simulink model "ULMPC_ES_multi_sine"  (R2020a)
settings: Solver=ode1  StartTime=0.0  StopTime=1900  FixedStep=1/600  RelTol=1e-3
values from neighbouring files (symbols this model uses):
  alpha_IC = [60000;10000]    [initial_run.m]
  amp = 0.03*[60000;10000]    [initial_run.m]
  freq = [(2*pi)/(5*Tr); (2*pi)/(4*Tr)]    [initial_run.m]
  gain_es = -[0.01;0.007]*30000    [initial_run.m]
  i_max = 0.85    [initial_run.m]
  Q = 16    [initial_run.m]
  R_weight = 10    [initial_run.m]
  Tr = 4    [initial_run.m]
  Ts = 0.01    [initial_run.m]
  Ts_ade = 0.01    [initial_run.m]
  Ts_es = 0.01    [initial_run.m]
  Z = 5    [initial_run.m]
undefined symbols (not defined in the file or in its folder): B, DiscIntNeverNeededParam, J, Km, N_ade, R, time, w_r
libraries: simulink x5, dspindex x2, dspstat3 x1
settings Model: Creator=Bryant Zhou  LastModifiedBy=Bryant Zhou

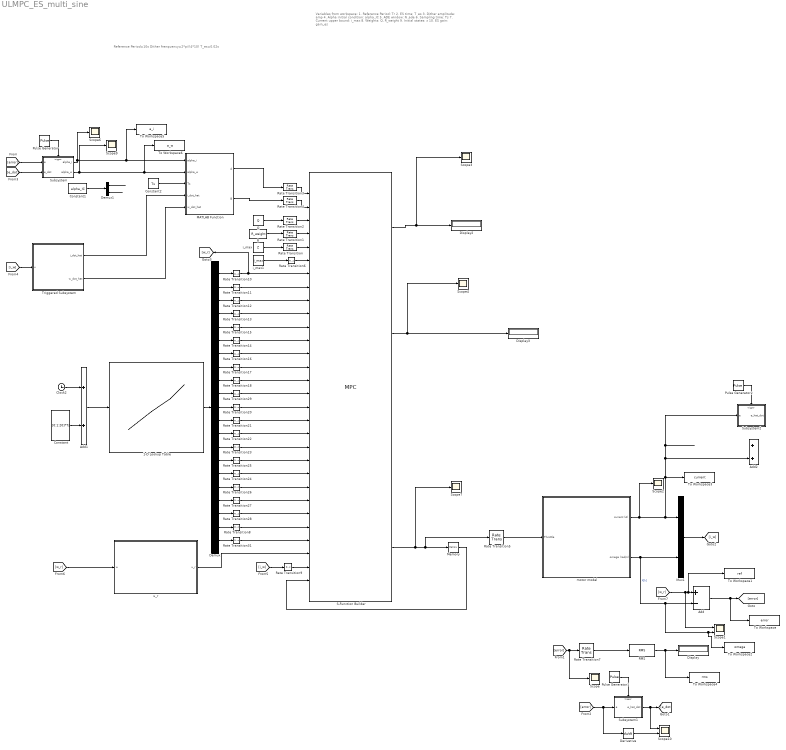
== system ULMPC_ES_multi_sine ==
  note: Variables from workspace:
      | 1. Reference Period: Tr
      | 2. ES time: T_es
      | 3. Dither amplitude: amp
      | 4. Alpha initial condition: alpha_IC
      | 5. ADE window: N_ade
      | 6. Sampling time: Ts
      | 7. Current upper bound: i_max
      | 8. Weights: Q, R_weight
      | 9. Initial states: x
      | 10. ES gain: gain_es
  note: Reference Period=10s
      | Dither frenquency=2*pi/(4*10)
      | T_es=0.02s
  1-D Lookup Table : Lookup_n-D  NumberOfTableDimensions=1  BreakpointsForDimension1=time  Table=w_r  InternalRulePriority=Speed  RndMeth=Simplest  InputSameDT=on
  Add : Sum  Inputs=+-
  Add1 : Sum
  Add2 : Sum
  Clock2 : Clock
  Constant : Constant  Value=[0:1:20]*Ts
  Constant1 : Constant  Value=alpha_IC
  Constant2 : Constant  Value=Ts
  Demux : Demux  Outputs=21
  Demux1 : Demux  Outputs=2
  Derivative : Derivative
  Display : Display
  Display2 : Display
  Display3 : Display
  MATLAB Function : MATLAB Function  TreatAsAtomicUnit=on
  Memory : Memory  InheritSampleTime=on
  Mux1 : Mux  Inputs=2
  Pulse Generator : DiscretePulseGenerator  PulseType=Time based  Period=Ts_es  PulseWidth=50
  Pulse Generator1 : DiscretePulseGenerator  PulseType=Time based  Period=Ts_ade  PulseWidth=50
  Pulse Generator2 : DiscretePulseGenerator  PulseType=Time based  Period=Ts_ade  PulseWidth=50
  Q : Constant  Value=Q
  R : Constant  Value=R_weight
  RMS : dspstat3/RMS  run=on  directionMode=Entire input  dimension=1  reset_popup=None
  Rate Transition{,1..18,20..29,31} (30 alike) : RateTransition
  S-Function Builder : S-Function  InitFcn=try, set_param(gcb,'FunctionName','MPC'), end  FunctionName=MPC  SFunctionModules=MPC_wrapper solver util matrix_support ldl  SFunctionDeploymentMode=off  EnableBusSupport=off  mask(S-Function Builder){}
      mask help: Simulink:masks:SFunctionBuilder_MD
      mask init:
      | val = [[.9  0.75 0.75 1 1 .9 .9 1]',[1 1 0.75 0.75 .9 .9 1 .9]'];try , sys = get_param(gcb,'SfunBuilderFcnName');if isempty(sys), sys = get_param(gcb,'FunctionName'); end,catch, sys = get_param(gcb,'FunctionName'); end
      settings: CopyFcn=set_param(gcbh,'LinkStatus','none')  PreSaveFcn=try, set_param(gcb,'FunctionName','MPC'), end  OpenFcn=sfunctionwizard(gcbh)
      mask Display: plot(val(:,1),val(:,2)),disp(sys), port_label('input',1,'A'), port_label('input',2,'B'), port_label('input',3,'Q'), port_label('input',4,'R'), port_label('input',5,'Z'), port_label('input',6,'i_max'), port_label('input',7,'w_r_0'), port_label('input',8,'w_r_1'), port_label('input',9,'w_r_2'), port_label('input',10,'w_r_3'), port_label('input',11,'w_r_4'), port_label('input',12,'w_r_5'), port_label('input',13,'w_r_6'), port_label('input',14,'w_r_7'), port_label('input',15,'w_r_8'), port_label('input',16,'w_r_9'), port_label('input',17,'w_r_10'), port_label('input',18,'w_r_11'), port_label('input',19,'w_r_12'), port_label('input',20,'w_r_13'), port_label('input',21,'w_r_14'), port_label('input',22,'w_r_15'), port_label('input',23,'w_r_16'), port_label('input',24,'w_r_17'), port_label('input',25,'w_r_18'), port_label('input',26,'w_r_19'), port_label('input',27,'w_r_20'), port_label('input',28,'u_r'), port_label('input',29,'x_0'), port_label('input',30,'th_last'), port_label('output',1,'th_delta'), port_label('output',2,'i'), port_label('output',3,'omega'), port_label('output',4,'th_opt')
  Scope{,2..4,6..7,9} (7 alike) : Scope
  Scope1 : Scope  NumInputPorts=2
  Scope10 : Scope  NumInputPorts=2
  Subsystem : Subsystem
  Subsystem1 : Subsystem
  Subsystem2 : Subsystem
  To Workspace : ToWorkspace  VariableName=error  SaveFormat=Timeseries  SampleTime=-1
  To Workspace1 : ToWorkspace  VariableName=ref  SaveFormat=Timeseries  SampleTime=-1
  To Workspace2 : ToWorkspace  VariableName=omega  SaveFormat=Timeseries  SampleTime=-1
  To Workspace3 : ToWorkspace  VariableName=current  SaveFormat=Timeseries  SampleTime=-1
  To Workspace4 : ToWorkspace  VariableName=rms  SaveFormat=Timeseries  SampleTime=-1
  To Workspace5 : ToWorkspace  VariableName=a_i  SaveFormat=Timeseries  SampleTime=-1
  To Workspace6 : ToWorkspace  VariableName=a_w  SaveFormat=Timeseries  SampleTime=-1
  Triggered Subsystem : Subsystem  TreatAsAtomicUnit=on
  i_max : Constant  Value=Z
  i_max1 : Constant  Value=i_max
  motor model : Subsystem
  u_r : Subsystem
  wires:
  Rate Transition/1 -> S-Function Builder/5
  i_max/1 -> Rate Transition/1
  Rate Transition1/1 -> S-Function Builder/4
  Rate Transition2/1 -> S-Function Builder/3
  R/1 -> Rate Transition1/1
  Q/1 -> Rate Transition2/1
  Subsystem/2(alpha_w) -> Scope9/1, To Workspace6/1, MATLAB Function/2(alpha_w)
  Rate Transition3/1 -> S-Function Builder/1
  Rate Transition4/1 -> S-Function Builder/2
  MATLAB Function/1(A) -> Rate Transition3/1
  MATLAB Function/2(B) -> Rate Transition4/1
  S-Function Builder/2 -> Scope4/1, Display3/1
  motor model/2(omega (rad/s)) -> Mux1/2, To Workspace2/1, Scope1/2, Add/2  "X[k]"
  i_max1/1 -> Rate Transition6/1
  S-Function Builder/4 -> Scope7/1, Rate Transition5/1, Memory/1
  Memory/1 -> S-Function Builder/30
  S-Function Builder/1 -> Scope3/1, Display2/1
  Constant2/1 -> MATLAB Function/3(Ts)
  Rate Transition6/1 -> S-Function Builder/6
  Rate Transition10/1 -> [w_r], S-Function Builder/7
  Rate Transition11/1 -> S-Function Builder/8
  Rate Transition12/1 -> S-Function Builder/9
  Rate Transition13/1 -> S-Function Builder/10
  Rate Transition14/1 -> S-Function Builder/12
  Rate Transition15/1 -> S-Function Builder/11
  Rate Transition16/1 -> S-Function Builder/13
  Rate Transition17/1 -> S-Function Builder/14
  Rate Transition18/1 -> S-Function Builder/15
  Rate Transition28/1 -> S-Function Builder/25
  Rate Transition27/1 -> S-Function Builder/24
  Rate Transition26/1 -> S-Function Builder/23
  Rate Transition25/1 -> S-Function Builder/21
  Rate Transition24/1 -> S-Function Builder/22
  Rate Transition23/1 -> S-Function Builder/20
  Rate Transition22/1 -> S-Function Builder/19
  Rate Transition21/1 -> S-Function Builder/18
  Rate Transition20/1 -> S-Function Builder/17
  Rate Transition29/1 -> S-Function Builder/16
  Rate Transition9/1 -> S-Function Builder/29
  Rate Transition5/1 -> motor model/1(Throttle)
  [i_w] -> Rate Transition9/1
  Subsystem/1(alpha_i) -> MATLAB Function/1(alpha_i), To Workspace5/1, Scope6/1
  Constant1/1 -> Demux1/1
  [error] -> Subsystem/1(e)
  RMS/1 -> To Workspace4/1, Display/1
  Rate Transition7/1 -> RMS/1
  Add/1 -> To Workspace/1, [error]
  Add1/1 -> 1-D Lookup Table/1
  Clock2/1 -> Add1/1
  1-D Lookup Table/1 -> Demux/1
  Constant/1 -> Add1/2
  Rate Transition8/1 -> S-Function Builder/26
  Rate Transition31/1 -> S-Function Builder/27
  u_r/1(u_r) -> S-Function Builder/28
  Triggered Subsystem/1(i_dot_hat) -> MATLAB Function/4(i_dot_hat)
  Triggered Subsystem/2(w_dot_hat) -> MATLAB Function/5(w_dot_hat)
  Pulse Generator/1 -> Subsystem/Trigger
  [error] -> Scope/1, Rate Transition7/1
  [e_dot] -> Subsystem/2(e_dot)
  [error] -> Derivative/1, Subsystem1/1(e)
  Subsystem1/1(e_hat_dot) -> Scope10/1, [e_dot]
  Pulse Generator1/1 -> Subsystem1/Trigger
  Derivative/1 -> Scope10/2
  Mux1/1 -> [i_w]
  [i_w] -> Triggered Subsystem/1(u)
  Demux/1 -> Rate Transition10/1
  Demux/2 -> Rate Transition11/1
  Demux/3 -> Rate Transition12/1
  Demux/4 -> Rate Transition13/1
  Demux/5 -> Rate Transition15/1
  Demux/6 -> Rate Transition14/1
  Demux/7 -> Rate Transition16/1
  Demux/8 -> Rate Transition17/1
  Demux/9 -> Rate Transition18/1
  Demux/10 -> Rate Transition29/1
  Demux/11 -> Rate Transition20/1
  Demux/12 -> Rate Transition21/1
  Demux/13 -> Rate Transition22/1
  Demux/14 -> Rate Transition23/1
  Demux/15 -> Rate Transition25/1
  Demux/16 -> Rate Transition24/1
  Demux/17 -> Rate Transition26/1
  Demux/18 -> Rate Transition27/1
  Demux/19 -> Rate Transition28/1
  Demux/20 -> Rate Transition8/1
  Demux/21 -> Rate Transition31/1
  [w_r] -> u_r/1(w)
  [w_r] -> Scope1/1, To Workspace1/1, Add/1
  Demux1/1 -> ?
  Demux1/2 -> ?
  motor model/1(current (A)) -> Scope2/1, Subsystem2/1(e), Add2/2, To Workspace3/1, Mux1/1
  Pulse Generator2/1 -> Subsystem2/Trigger

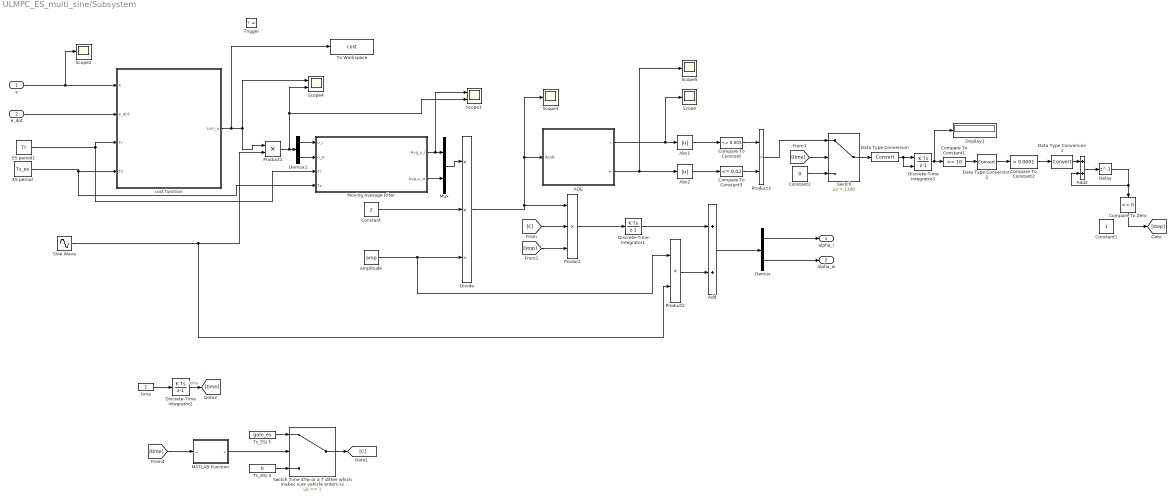
== system ULMPC_ES_multi_sine/Subsystem ==
  e : Inport
  e_dot : Inport  Port=2
  Trigger : TriggerPort  VariantControl=Variant  PortDimensions=1
  "ADE " : Subsystem
  Abs1 : Abs
  Abs2 : Abs
  Add : Sum
  Add2 : Sum
  Compare To Constant : simulink/Logic and Bit Operations/Compare To Constant  relop=<=  const=0.003  OutDataTypeStr=boolean
  Compare To Constant1 : simulink/Logic and Bit Operations/Compare To Constant  relop=>=  const=10  OutDataTypeStr=boolean
  Compare To Constant2 : simulink/Logic and Bit Operations/Compare To Constant  relop=>  const=0.0001  OutDataTypeStr=boolean
  Compare To Constant3 : simulink/Logic and Bit Operations/Compare To Constant  relop=<=  const=0.02  OutDataTypeStr=boolean
  Compare To Zero : simulink/Logic and Bit Operations/Compare To Zero  relop=<=  OutDataTypeStr=boolean
  Constant : Constant  Value=2
  Constant1 : Constant
  Constant2 : Constant  Value=0
  Data Type Conversion : DataTypeConversion
  Data Type Conversion1 : DataTypeConversion
  Data Type Conversion2 : DataTypeConversion
  Delay : Delay  DelayLength=1  InitialCondition=0
  Demux : Demux  Outputs=2
  Demux1 : Demux  Outputs=2
  Discrete-Time Integrator1 : DiscreteIntegrator  InitialCondition=alpha_IC  SampleTime=-1  ICPrevOutput=DiscIntNeverNeededParam  ICPrevScaledInput=DiscIntNeverNeededParam
  Discrete-Time Integrator2 : DiscreteIntegrator  SampleTime=-1  ICPrevOutput=DiscIntNeverNeededParam  ICPrevScaledInput=DiscIntNeverNeededParam
  Discrete-Time Integrator3 : DiscreteIntegrator  ExternalReset=falling  SampleTime=-1  ICPrevOutput=DiscIntNeverNeededParam  ICPrevScaledInput=DiscIntNeverNeededParam
  Display1 : Display
  Divide : Product  Inputs=**/
  ES period : Constant  Value=Ts_es
  ES period1 : Constant  Value=Tr
  MATLAB Function : MATLAB Function  TreatAsAtomicUnit=on
  Moving Average Filter : MATLAB Function  TreatAsAtomicUnit=on
  Mux : Mux  Inputs=2
  Product : Product  Inputs=3
  Product1 : Product
  Product2 : Product
  Product3 : Product
  Scope{,2..3,5} (4 alike) : Scope
  Scope1 : Scope  NumInputPorts=2
  Scope4 : Scope  NumInputPorts=2
  Sine Wave : Sin  Frequency=freq
  Switch : Switch  Criteria=u2 > Threshold  Threshold=1100
  Switch Time 4Tw or a T dither which makes sure vehicle enters ss : Switch  Threshold=1
  To Workspace : ToWorkspace  VariableName=cost  SaveFormat=Timeseries  SampleTime=-1
  Ts_ES/ 3 : Constant  Value=0
  Ts_ES/ 5 : Constant  Value=gain_es
  amplitude : Constant  Value=amp
  cost function : MATLAB Function  TreatAsAtomicUnit=on
  time : Constant
  alpha_i : Outport
  alpha_w : Outport  Port=2
  wires:
  Demux/2 -> alpha_w/1
  Sine Wave/1 -> Product2/2, Product1/2
  Product/1 -> Discrete-Time Integrator1/1
  Add/1 -> Demux/1
  Product2/1 -> Add/2
  Discrete-Time Integrator1/1 -> Add/1
  Divide/1 -> Scope3/1, "ADE "/1(de/dt), Product/1
  [C] -> Product/2
  Product1/1 -> Scope4/2, Scope1/2, Demux1/1
  ES period1/1 -> Moving Average Filter/3(Tr), cost function/3(Tr)
  ES period/1 -> Moving Average Filter/4(Ts), cost function/4(Ts)
  Demux/1 -> alpha_i/1
  Constant/1 -> Divide/2
  e/1 -> cost function/1(e), Scope2/1
  Demux1/1 -> Moving Average Filter/1(u_i)
  Demux1/2 -> Moving Average Filter/2(u_w)
  Moving Average Filter/1(Avg_u_i) -> Scope1/1, Mux/1
  Moving Average Filter/2(Avg_u_w) -> Mux/2
  Mux/1 -> Divide/1
  amplitude/1 -> Product2/1, Divide/3
  cost function/1(sum_u) -> To Workspace/1, Product1/1, Scope4/1
  "ADE "/1(i) -> Abs1/1, Scope/1
  time/1 -> Discrete-Time Integrator2/1
  Switch Time 4Tw or a T dither which makes sure vehicle enters ss/1 -> [C]
  Ts_ES/ 3/1 -> Switch Time 4Tw or a T dither which makes sure vehicle enters ss/3
  Ts_ES/ 5/1 -> Switch Time 4Tw or a T dither which makes sure vehicle enters ss/1
  e_dot/1 -> cost function/2(e_dot)
  Compare To Constant1/1 -> Data Type Conversion2/1
  Data Type Conversion/1 -> Discrete-Time Integrator3/2, Discrete-Time Integrator3/1
  Discrete-Time Integrator3/1 -> Display1/1, Compare To Constant1/1
  Abs1/1 -> Compare To Constant/1
  Compare To Constant2/1 -> Data Type Conversion1/1
  Delay/1 -> Compare To Zero/1, Add2/2
  Data Type Conversion2/1 -> Compare To Constant2/1
  Data Type Conversion1/1 -> Add2/1
  Add2/1 -> Delay/1
  "ADE "/2(w) -> Scope5/1, Abs2/1
  Abs2/1 -> Compare To Constant3/1
  Compare To Constant/1 -> Product3/1
  Compare To Constant3/1 -> Product3/2
  [stop] -> Product/3
  Constant2/1 -> Switch/3
  Switch/1 -> Data Type Conversion/1
  [time] -> Switch/2
  Product3/1 -> Switch/1
  Discrete-Time Integrator2/1 -> [time]  "time"
  MATLAB Function/1(y) -> Switch Time 4Tw or a T dither which makes sure vehicle enters ss/2
  Compare To Zero/1 -> [stop]
  [time] -> MATLAB Function/1(u)

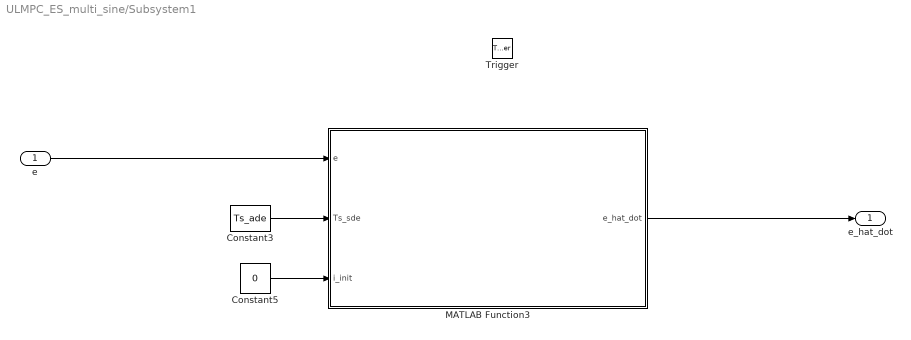
== system ULMPC_ES_multi_sine/Subsystem1 ==
  e : Inport
  Trigger : TriggerPort  VariantControl=Variant  PortDimensions=1
  Constant3 : Constant  Value=Ts_ade
  Constant5 : Constant  Value=0
  MATLAB Function3 : MATLAB Function  TreatAsAtomicUnit=on
  e_hat_dot : Outport
  wires:
  Constant5/1 -> MATLAB Function3/3(i_init)
  Constant3/1 -> MATLAB Function3/2(Ts_sde)
  e/1 -> MATLAB Function3/1(e)
  MATLAB Function3/1(e_hat_dot) -> e_hat_dot/1

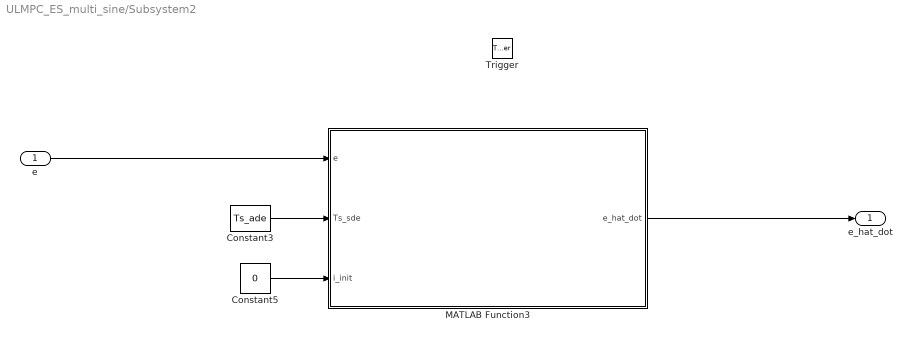
== system ULMPC_ES_multi_sine/Subsystem2 ==
  e : Inport
  Trigger : TriggerPort  VariantControl=Variant  PortDimensions=1
  Constant3 : Constant  Value=Ts_ade
  Constant5 : Constant  Value=0
  MATLAB Function3 : MATLAB Function  TreatAsAtomicUnit=on
  e_hat_dot : Outport
  wires:
  Constant5/1 -> MATLAB Function3/3(i_init)
  Constant3/1 -> MATLAB Function3/2(Ts_sde)
  e/1 -> MATLAB Function3/1(e)
  MATLAB Function3/1(e_hat_dot) -> e_hat_dot/1

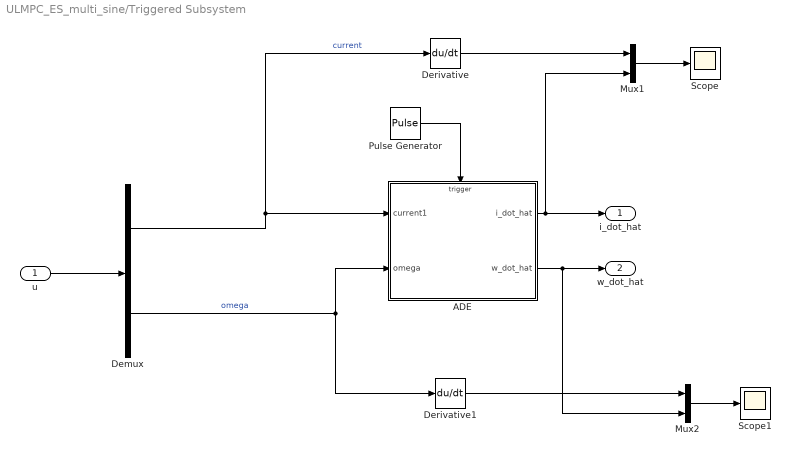
== system ULMPC_ES_multi_sine/Triggered Subsystem ==
  u : Inport
  "ADE " : Subsystem
  Demux : Demux  Outputs=2
  Derivative : Derivative
  Derivative1 : Derivative
  Mux1 : Mux  Inputs=2
  Mux2 : Mux  Inputs=2
  Pulse Generator : DiscretePulseGenerator  PulseType=Time based  Period=Ts_ade  PulseWidth=50
  Scope : Scope
  Scope1 : Scope
  i_dot_hat : Outport
  w_dot_hat : Outport  Port=2
  wires:
  Demux/1 -> "ADE "/1(current1), Derivative/1  "current"
  Demux/2 -> "ADE "/2(omega), Derivative1/1  "omega"
  "ADE "/2(w_dot_hat) -> Mux2/2, w_dot_hat/1
  Derivative/1 -> Mux1/1
  Mux1/1 -> Scope/1
  u/1 -> Demux/1
  Mux2/1 -> Scope1/1
  Derivative1/1 -> Mux2/1
  Pulse Generator/1 -> "ADE "/Trigger
  "ADE "/1(i_dot_hat) -> Mux1/2, i_dot_hat/1

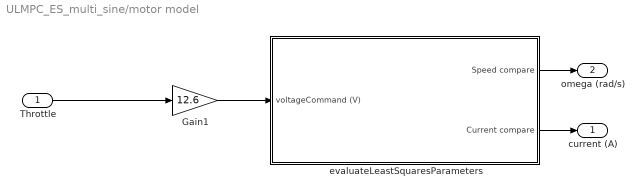
== system ULMPC_ES_multi_sine/motor model ==
  Throttle : Inport
  Gain1 : Gain  Gain=12.6
  evaluateLeastSquaresParameters : Subsystem
  current (A) : Outport
  omega (rad/s) : Outport  Port=2
  wires:
  Gain1/1 -> evaluateLeastSquaresParameters/1(voltageCommand (V))
  Throttle/1 -> Gain1/1
  evaluateLeastSquaresParameters/2(Current compare) -> current (A)/1
  evaluateLeastSquaresParameters/1(Speed compare) -> omega (rad/s)/1

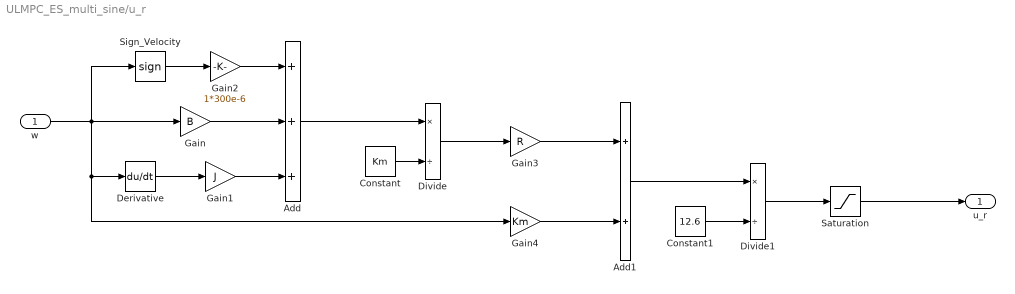
== system ULMPC_ES_multi_sine/u_r ==
  w : Inport
  Add : Sum  Inputs=+++
  Add1 : Sum
  Constant : Constant  Value=Km
  Constant1 : Constant  Value=12.6
  Derivative : Derivative
  Divide : Product  Inputs=*/
  Divide1 : Product  Inputs=*/
  Gain : Gain  Gain=B
  Gain1 : Gain  Gain=J
  Gain2 : Gain  Gain=1*300e-6
  Gain3 : Gain  Gain=R
  Gain4 : Gain  Gain=Km
  Saturation : Saturate  UpperLimit=1  LowerLimit=-1
  Sign_Velocity : Signum
  u_r : Outport
  wires:
  w/1 -> Gain/1, Sign_Velocity/1, Derivative/1, Gain4/1
  Gain/1 -> Add/2
  Derivative/1 -> Gain1/1
  Gain1/1 -> Add/3
  Gain2/1 -> Add/1
  Sign_Velocity/1 -> Gain2/1
  Add/1 -> Divide/1
  Constant/1 -> Divide/2
  Divide/1 -> Gain3/1
  Gain3/1 -> Add1/1
  Gain4/1 -> Add1/2
  Add1/1 -> Divide1/1
  Constant1/1 -> Divide1/2
  Divide1/1 -> Saturation/1
  Saturation/1 -> u_r/1

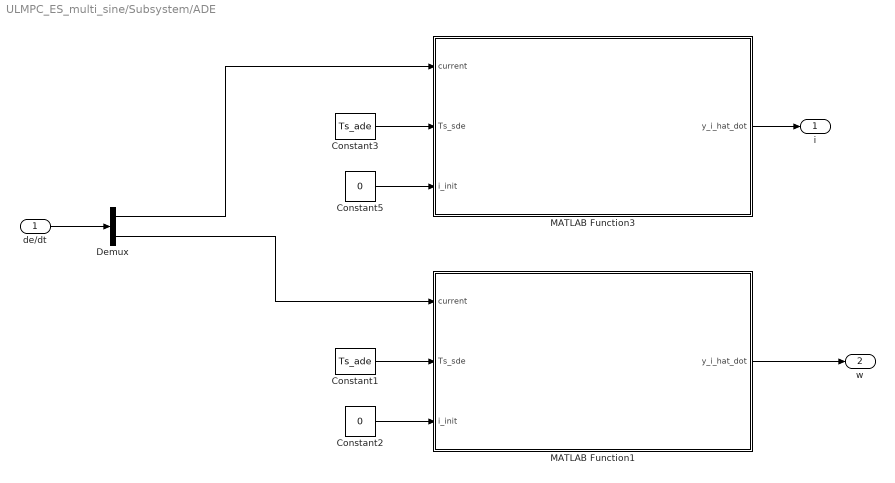
== system ULMPC_ES_multi_sine/Subsystem/ADE  ==
  de/dt : Inport
  Constant1 : Constant  Value=Ts_ade
  Constant2 : Constant  Value=0
  Constant3 : Constant  Value=Ts_ade
  Constant5 : Constant  Value=0
  Demux : Demux  Outputs=2
  MATLAB Function1 : MATLAB Function  TreatAsAtomicUnit=on
  MATLAB Function3 : MATLAB Function  TreatAsAtomicUnit=on
  i : Outport  VectorParamsAs1DForOutWhenUnconnected=off
  w : Outport  Port=2  VectorParamsAs1DForOutWhenUnconnected=off
  wires:
  Constant5/1 -> MATLAB Function3/3(i_init)
  Constant3/1 -> MATLAB Function3/2(Ts_sde)
  Demux/2 -> MATLAB Function1/1(current)
  Constant1/1 -> MATLAB Function1/2(Ts_sde)
  Constant2/1 -> MATLAB Function1/3(i_init)
  de/dt/1 -> Demux/1
  Demux/1 -> MATLAB Function3/1(current)
  MATLAB Function3/1(y_i_hat_dot) -> i/1
  MATLAB Function1/1(y_i_hat_dot) -> w/1

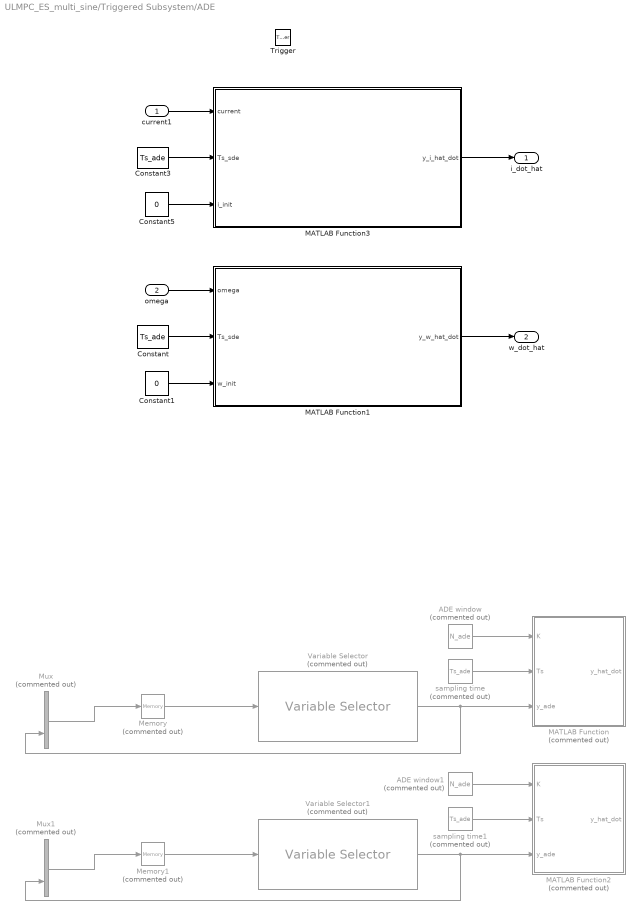
== system ULMPC_ES_multi_sine/Triggered Subsystem/ADE  ==
  current1 : Inport
  omega : Inport  Port=2
  Trigger : TriggerPort  VariantControl=Variant  PortDimensions=1
  ADE window : Constant  Commented=on  Value=N_ade
  ADE window1 : Constant  Commented=on  Value=N_ade
  Constant : Constant  Value=Ts_ade
  Constant1 : Constant  Value=0
  Constant3 : Constant  Value=Ts_ade
  Constant5 : Constant  Value=0
  MATLAB Function : MATLAB Function  Commented=on  TreatAsAtomicUnit=on
  MATLAB Function1 : MATLAB Function  TreatAsAtomicUnit=on
  MATLAB Function2 : MATLAB Function  Commented=on  TreatAsAtomicUnit=on
  MATLAB Function3 : MATLAB Function  TreatAsAtomicUnit=on
  Memory : Memory  Commented=on  InheritSampleTime=on
  Memory1 : Memory  Commented=on  InheritSampleTime=on
  Mux : Mux  Commented=on  Inputs=2
  Mux1 : Mux  Commented=on  Inputs=2
  Variable Selector : dspindex/Variable Selector  Commented=on  NumInputs=1  rowsOrCols=Rows  IdxMode=Fixed  Elements=1:5  ZerOneIdxMode=One-based  errmode=Clip Index  FillMode=on  FillValues=0
  Variable Selector1 : dspindex/Variable Selector  Commented=on  NumInputs=1  rowsOrCols=Rows  IdxMode=Fixed  Elements=1:5  ZerOneIdxMode=One-based  errmode=Clip Index  FillMode=on  FillValues=0
  sampling time : Constant  Commented=on  Value=Ts_ade
  sampling time1 : Constant  Commented=on  Value=Ts_ade
  i_dot_hat : Outport  VectorParamsAs1DForOutWhenUnconnected=off
  w_dot_hat : Outport  Port=2  VectorParamsAs1DForOutWhenUnconnected=off
  wires:
  omega/1 -> MATLAB Function1/1(omega)
  MATLAB Function1/1(y_w_hat_dot) -> w_dot_hat/1
  Constant/1 -> MATLAB Function1/2(Ts_sde)
  Constant1/1 -> MATLAB Function1/3(w_init)
  sampling time/1 -> MATLAB Function/2(Ts)
  Mux/1 -> Memory/1
  ADE window/1 -> MATLAB Function/1(K)
  Memory/1 -> Variable Selector/1
  Variable Selector/1 -> Mux/2, MATLAB Function/3(y_ade)
  sampling time1/1 -> MATLAB Function2/2(Ts)
  Mux1/1 -> Memory1/1
  ADE window1/1 -> MATLAB Function2/1(K)
  Memory1/1 -> Variable Selector1/1
  Variable Selector1/1 -> Mux1/2, MATLAB Function2/3(y_ade)
  Constant5/1 -> MATLAB Function3/3(i_init)
  Constant3/1 -> MATLAB Function3/2(Ts_sde)
  MATLAB Function3/1(y_i_hat_dot) -> i_dot_hat/1
  current1/1 -> MATLAB Function3/1(current)

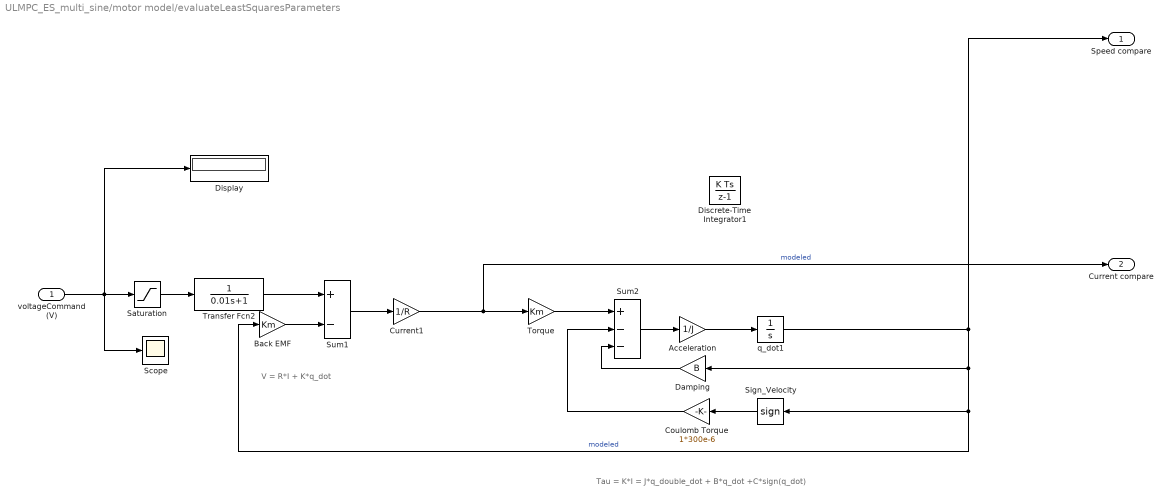
== system ULMPC_ES_multi_sine/motor model/evaluateLeastSquaresParameters ==
  note: Tau = K*I = J*q_double_dot + B*q_dot +C*sign(q_dot)
  note: V = R*I + K*q_dot
  voltageCommand (V) : Inport
  Acceleration : Gain  Gain=1/J
  Back EMF : Gain  Gain=Km
  Coulomb Torque : Gain  Gain=1*300e-6
  Current1 : Gain  Gain=1/R
  Damping : Gain  Gain=B
  Discrete-Time Integrator1 : DiscreteIntegrator  SampleTime=-1  ICPrevOutput=DiscIntNeverNeededParam  ICPrevScaledInput=DiscIntNeverNeededParam
  Display : Display
  Saturation : Saturate  UpperLimit=12.6  LowerLimit=-12.6
  Scope : Scope
  Sign_Velocity : Signum
  Sum1 : Sum  Inputs=+-
  Sum2 : Sum  Inputs=+--
  Torque : Gain  Gain=Km
  Transfer Fcn2 : TransferFcn  Denominator=[0.01 1]
  q_dot1 : Integrator
  Speed compare : Outport
  Current compare : Outport  Port=2
  wires:
  q_dot1/1 -> Speed compare/1, Sign_Velocity/1, Back EMF/1, Damping/1  "modeled"
  Current1/1 -> Current compare/1, Torque/1  "modeled"
  Damping/1 -> Sum2/3
  Sum2/1 -> Acceleration/1
  Coulomb Torque/1 -> Sum2/2
  Acceleration/1 -> q_dot1/1
  Sign_Velocity/1 -> Coulomb Torque/1
  Back EMF/1 -> Sum1/2
  voltageCommand (V)/1 -> Scope/1, Display/1, Saturation/1
  Sum1/1 -> Current1/1
  Torque/1 -> Sum2/1
  Saturation/1 -> Transfer Fcn2/1
  Transfer Fcn2/1 -> Sum1/1

== matlab function ULMPC_ES_multi_sine/Subsystem/Moving Average Filter ==
  settings: updateMethod=DISCRETE
  data: u_i input; u_w input; Avg_u_i output; Tr input; Ts input; Avg_u_w output
function [Avg_u_i,Avg_u_w]  = Moving_Average_For_Dither_Period(u_i, u_w, Tr,Ts)

    Ni = round(4*Tr/Ts);
    Nw = round(5*Tr/Ts);

    persistent x y;
    if isempty(x)
        x = zeros(Ni,1);
    end
    
    if isempty(y)
        y = zeros(Nw,1);
    end
    
    x = [u_i; x(1:end-1)];
    y = [u_w; y(1:end-1)];
    
    Avg_u_i = mean(x);
    Avg_u_w = mean(y);
    
end

== matlab function ULMPC_ES_multi_sine/Subsystem/cost function ==
  settings: updateMethod=DISCRETE
  data: e input; e_dot input; sum_u output; Tr input; Ts input
function sum_u  = cost_function(e, e_dot,Tr , Ts)

    N = round(Tr/Ts);
% 
%     persistent y;
%     if isempty(y)
%         y = zeros(N,1);
%     end
%     
%     y = [u; y(1:end-1)];
%     
%     sum_u = sum(y);
    % Initialization two vectors with Zero
    persistent y;
    if isempty(y)
        y = 0*ones(N+1,1);
    end
   
%% Update the two vectors with newly coming elements    
    y     = [e^2+e_dot^2;         y(1:end-1)];
   
    T = Ts*N;
    alpha = zeros(1,N+1);
    
    for k = 1:N+1
        if((k==1)||(k==N+1))
            alpha(k) = Ts/2;
        else
            alpha(k) = Ts;
        end
    end
    
    J_ev = alpha*y;
 
    sum_u  = J_ev/T;
end

== matlab function ULMPC_ES_multi_sine/Subsystem1/MATLAB Function3 ==
  settings: updateMethod=DISCRETE
  data: e input; e_hat_dot output; Ts_sde input; i_init input
function e_hat_dot  = buffer(e,Ts_sde, i_init)
    N = 10;
    %Ts = 0.01;
    persistent y;
    
    if isempty(y)
        y=i_init*ones(N+1,1);
    end
    
    y = [e;y(1:end-1)];
    T = Ts_sde*N;
    P = zeros(1,N+1);
    P_alpha = P;
    for k = 1:N+1
        tao_k = (k-1)*Ts_sde;
        P(k) = T-2*tao_k;
        if((k==1)||(k==N+1))
            P_alpha(k) = P(k)*Ts_sde/2;
        else
            P_alpha(k) = P(k)*Ts_sde;
        end
    end
    
    e_hat_dot = P_alpha*y*6/(T^3);
end

== matlab function ULMPC_ES_multi_sine/MATLAB Function ==
  data: alpha_i input; A output; alpha_w input; B output; Ts input; i_dot_hat input; w_dot_hat input
function [A,B] = fcn(alpha_i, alpha_w, Ts, i_dot_hat, w_dot_hat)
A = [i_dot_hat*Ts;
    (w_dot_hat+alpha_w*Ts*i_dot_hat)*Ts];
B = [alpha_i*Ts;
    alpha_w*alpha_i*Ts*Ts];

== matlab function ULMPC_ES_multi_sine/Triggered Subsystem/ADE /MATLAB Function1 ==
  settings: updateMethod=DISCRETE
  data: omega input; Ts_sde input; w_init input; y_w_hat_dot output
function y_w_hat_dot  = buffer(omega,Ts_sde,w_init)
    N = 9;
    %Ts = 0.01;
    persistent y;
    if isempty(y)
        y=w_init*ones(N+1,1);%m/s
    end
 
    y = [omega;y(1:end-1)];
    T = Ts_sde*N;
    P = zeros(1,N+1);
    P_alpha = P;
    for k = 1:N+1
        tao_k = (k-1)*Ts_sde;
        P(k) = T-2*tao_k;
        if((k==1)||(k==N+1))
            P_alpha(k) = P(k)*Ts_sde/2;
        else
            P_alpha(k) = P(k)*Ts_sde;
        end
    end
    y_w_hat_dot = P_alpha*y*6/(T^3);
end

== matlab function ULMPC_ES_multi_sine/Subsystem/MATLAB Function ==
  data: u input; y output
function y = fcn(u)
if (u>100 && u<950) || u>1100
    y = 1;
else
    y = 0;
end

== matlab function ULMPC_ES_multi_sine/Subsystem2/MATLAB Function3 ==
  settings: updateMethod=DISCRETE
  data: e input; e_hat_dot output; Ts_sde input; i_init input
function e_hat_dot  = buffer(e,Ts_sde, i_init)
    N = 10;
    %Ts = 0.01;
    persistent y;
    
    if isempty(y)
        y=i_init*ones(N+1,1);
    end
    
    y = [e;y(1:end-1)];
    T = Ts_sde*N;
    P = zeros(1,N+1);
    P_alpha = P;
    for k = 1:N+1
        tao_k = (k-1)*Ts_sde;
        P(k) = T-2*tao_k;
        if((k==1)||(k==N+1))
            P_alpha(k) = P(k)*Ts_sde/2;
        else
            P_alpha(k) = P(k)*Ts_sde;
        end
    end
    
    e_hat_dot = P_alpha*y*6/(T^3);
end

== matlab function ULMPC_ES_multi_sine/Subsystem/ADE /MATLAB Function1 ==
  settings: updateMethod=DISCRETE
  data: current input; y_i_hat_dot output; Ts_sde input; i_init input
function y_i_hat_dot  = buffer(current,Ts_sde, i_init)
    N = 9;
    %Ts = 0.01;
    persistent y;
    
    if isempty(y)
        y=i_init*ones(N+1,1);
    end
    
    y = [current;y(1:end-1)];
    T = Ts_sde*N;
    P = zeros(1,N+1);
    P_alpha = P;
    for k = 1:N+1
        tao_k = (k-1)*Ts_sde;
        P(k) = T-2*tao_k;
        if((k==1)||(k==N+1))
            P_alpha(k) = P(k)*Ts_sde/2;
        else
            P_alpha(k) = P(k)*Ts_sde;
        end
    end
    
    y_i_hat_dot = P_alpha*y*6/(T^3);
end

== matlab function ULMPC_ES_multi_sine/Triggered Subsystem/ADE /MATLAB Function ==
  data: K input; y_hat_dot output size=[1]; Ts input; y_ade input
function y_hat_dot  = fcn(K,Ts,y_ade)
P = zeros(1,K+1);
Tade = K*Ts;
for i = 1:K+1
    Tk = (i-1)*Ts;
    if i == 1 || i == K+1
        a = Ts/2;
    else
        a = Ts;
    end    
    P(1,i) = a*6/(Tade^3)*(Tade-2*Tk);
end
y_hat_dot = P*y_ade;

== matlab function ULMPC_ES_multi_sine/Triggered Subsystem/ADE /MATLAB Function2 ==
  data: K input; y_hat_dot output size=[1]; Ts input; y_ade input
function y_hat_dot  = fcn(K,Ts,y_ade)
P = zeros(1,K+1);
Tade = K*Ts;
for i = 1:K+1
    Tk = (i-1)*Ts;
    if i == 1 || i == K+1
        a = Ts/2;
    else
        a = Ts;
    end    
    P(1,i) = a*6/(Tade^3)*(Tade-2*Tk);
end
y_hat_dot = P*y_ade;

== matlab function ULMPC_ES_multi_sine/Triggered Subsystem/ADE /MATLAB Function3 ==
  settings: updateMethod=DISCRETE
  data: current input; y_i_hat_dot output; Ts_sde input; i_init input
function y_i_hat_dot  = buffer(current,Ts_sde, i_init)
    N = 9;
    %Ts = 0.01;
    persistent y;
    
    if isempty(y)
        y=i_init*ones(N+1,1);
    end
    
    y = [current;y(1:end-1)];
    T = Ts_sde*N;
    P = zeros(1,N+1);
    P_alpha = P;
    for k = 1:N+1
        tao_k = (k-1)*Ts_sde;
        P(k) = T-2*tao_k;
        if((k==1)||(k==N+1))
            P_alpha(k) = P(k)*Ts_sde/2;
        else
            P_alpha(k) = P(k)*Ts_sde;
        end
    end
    
    y_i_hat_dot = P_alpha*y*6/(T^3);
end

== matlab function ULMPC_ES_multi_sine/Subsystem/ADE /MATLAB Function3 ==
  settings: updateMethod=DISCRETE
  data: current input; y_i_hat_dot output; Ts_sde input; i_init input
function y_i_hat_dot  = buffer(current,Ts_sde, i_init)
    N = 9;
    %Ts = 0.01;
    persistent y;
    
    if isempty(y)
        y=i_init*ones(N+1,1);
    end
    
    y = [current;y(1:end-1)];
    T = Ts_sde*N;
    P = zeros(1,N+1);
    P_alpha = P;
    for k = 1:N+1
        tao_k = (k-1)*Ts_sde;
        P(k) = T-2*tao_k;
        if((k==1)||(k==N+1))
            P_alpha(k) = P(k)*Ts_sde/2;
        else
            P_alpha(k) = P(k)*Ts_sde;
        end
    end
    
    y_i_hat_dot = P_alpha*y*6/(T^3);
end
